simulink model "N_WT"  (R2024b)
settings: Solver=VariableStepAuto  StartTime=0.0  StopTime=10.0  RelTol=1e-3
values from neighbouring files (symbols this model uses):
  Ga = -0.09    [P2.m]
  Gf = 1/(Gs*Kd)    (= 1)    [P2.m]
  Gs = 1    [P2.m]
libraries: cstblocks x2
settings Model: Creator=lucap  LastModifiedBy=lucap

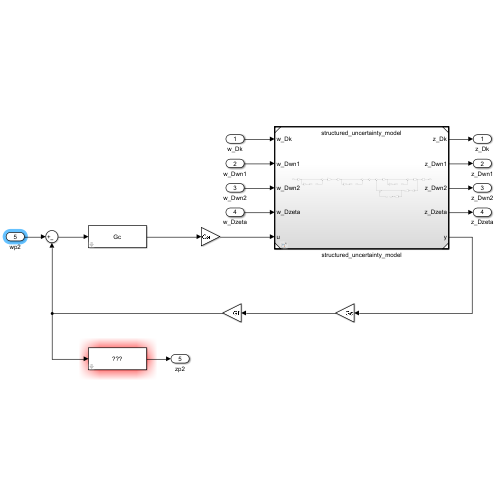
[thumbnail: Simulink's stored preview of the top-level diagram]
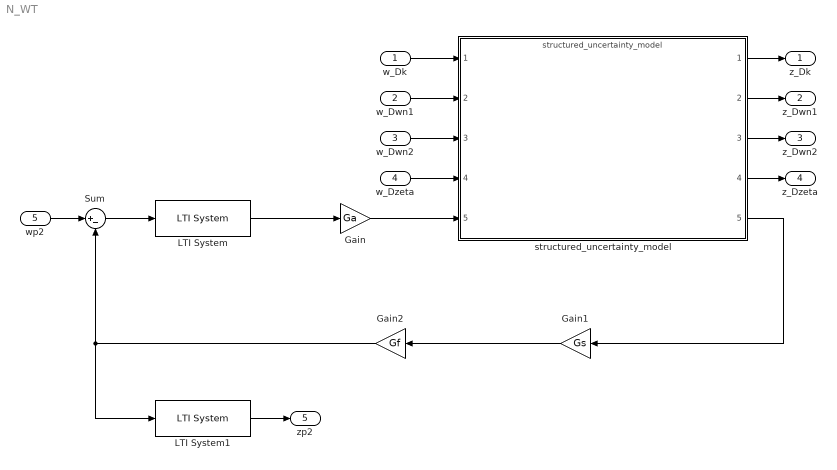
== system N_WT ==
  w_Dk : Inport
  w_Dwn1 : Inport  Port=2
  w_Dwn2 : Inport  Port=3
  w_Dzeta : Inport  Port=4
  wp2 : Inport  Port=5
  Gain : Gain  Gain=Ga
  Gain1 : Gain  Gain=Gs
  Gain2 : Gain  Gain=Gf
  LTI System : cstblocks/LTI System  sys=Gc  IC=[]  PadeOrder=0
  LTI System1 : cstblocks/LTI System  sys=WT_mu  IC=[]  PadeOrder=0
  Sum : Sum  Inputs=|+-
  structured_uncertainty_model : ModelReference  ModelNameDialog=structured_uncertainty_model.slx  SimulationMode=Normal  ModelReferenceVersion=1.4
  z_Dk : Outport
  z_Dwn1 : Outport  Port=2
  z_Dwn2 : Outport  Port=3
  z_Dzeta : Outport  Port=4
  zp2 : Outport  Port=5
  wires:
  structured_uncertainty_model/2 -> z_Dwn1/1
  w_Dk/1 -> structured_uncertainty_model/1
  structured_uncertainty_model/1 -> z_Dk/1
  structured_uncertainty_model/3 -> z_Dwn2/1
  structured_uncertainty_model/4 -> z_Dzeta/1
  LTI System/1 -> Gain/1
  Gain2/1 -> Sum/2, LTI System1/1
  w_Dwn1/1 -> structured_uncertainty_model/2
  wp2/1 -> Sum/1
  structured_uncertainty_model/5 -> Gain1/1
  LTI System1/1 -> zp2/1
  Sum/1 -> LTI System/1
  w_Dzeta/1 -> structured_uncertainty_model/4
  w_Dwn2/1 -> structured_uncertainty_model/3
  Gain/1 -> structured_uncertainty_model/5
  Gain1/1 -> Gain2/1
